simulink library "opm_grc"  (R2024a)
settings: Solver=VariableStepAuto  StartTime=0.0  StopTime=10.0  RelTol=1e-3
undefined symbols (not defined in the file or in its folder): ENUM_IVTROPMODE_ASCLO, ENUM_IVTROPMODE_DTCYCTRL, ENUM_IVTROPMODE_FW, ENUM_IVTROPMODE_IVTROFF, ENUM_MOTMOD_AFTERRUN, ENUM_MOTMOD_DISCHARGE, ENUM_MOTMOD_FAILURE, ENUM_MOTMOD_INIT, ENUM_MOTMOD_READY, ENUM_MOTMOD_SPDCTRL, ENUM_MOTMOD_STANDBY, ENUM_MOTMOD_TQCTROL, GRC_FAKE_SAMPLE_TIME, KOPM_IVTROpMode_enum_ovrdflg, KOPM_IVTROpMode_enum_ovrdval, KOPM_MotMod_enum_ovrdflg, KOPM_MotMod_enum_ovrdval, KOPM_PsvDischrgEna_flg_ovrdflg, KOPM_PsvDischrgEna_flg_ovrdval, OpMod_bDcha2AfterRunMor_C, OpMod_bService_C, OpMod_nRot2AfterRun_C, OpMod_nRotASCDi_C, OpMod_nRotASCEna_C, OpMod_ResolverEnt_C, OpMod_tiDcha2AfterRun_C, OpMod_uDCSide2AfterRun_C
libraries: GRC_Lib x1
settings Model: Creator=FVT22063  LastModifiedBy=FVT22063

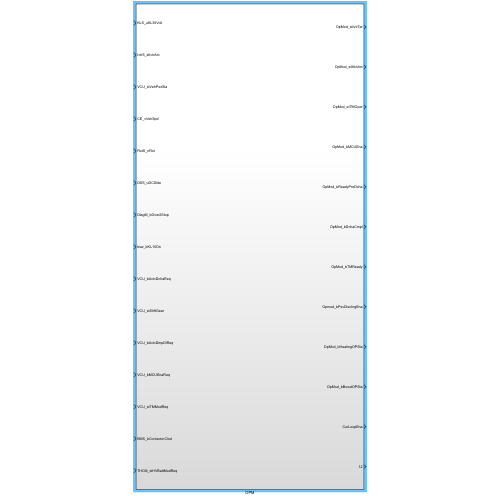
[thumbnail: Simulink's stored preview of the top-level diagram]
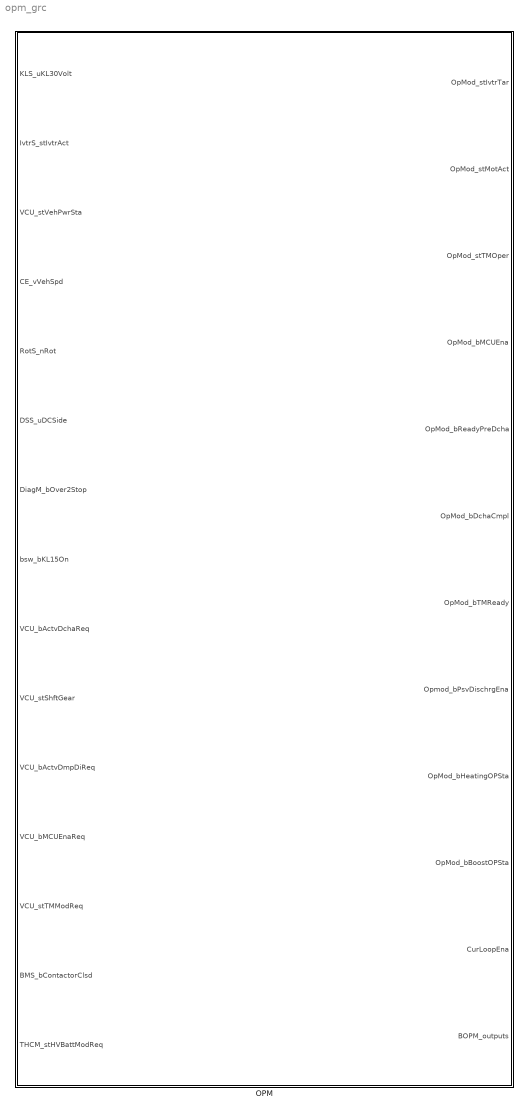
== system opm_grc ==
  OPM : Subsystem

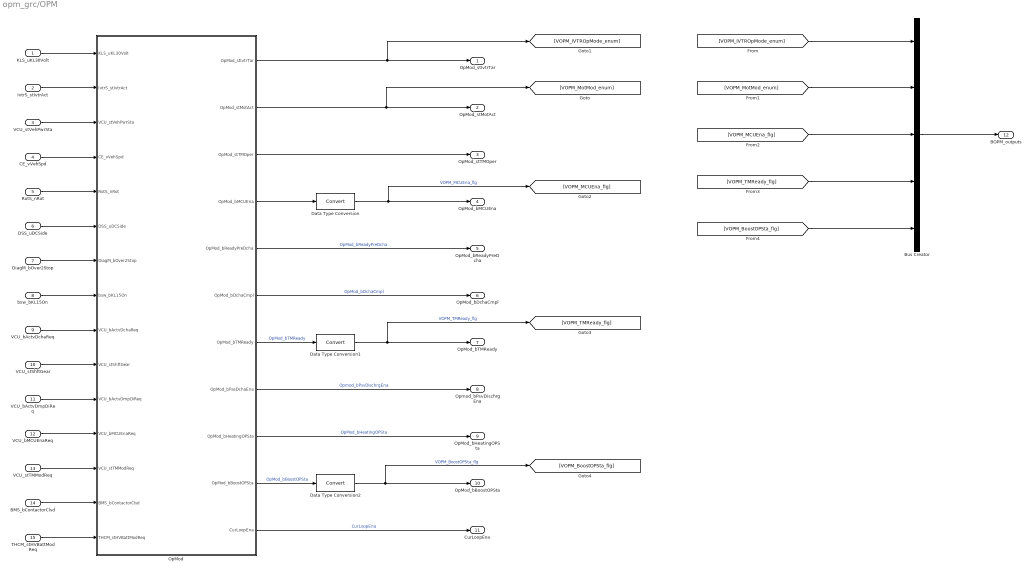
== system opm_grc/OPM ==
  KLS_uKL30Volt : Inport
  IvtrS_stIvtrAct : Inport  Port=2
  VCU_stVehPwrSta : Inport  Port=3
  CE_vVehSpd : Inport  Port=4
  RotS_nRot : Inport  Port=5
  DSS_uDCSide : Inport  Port=6
  DiagM_bOver2Stop : Inport  Port=7
  bsw_bKL15On : Inport  Port=8
  VCU_bActvDchaReq : Inport  Port=9
  VCU_stShftGear : Inport  Port=10
  VCU_bActvDmpDiReq : Inport  Port=11
  VCU_bMCUEnaReq : Inport  Port=12
  VCU_stTMModReq : Inport  Port=13
  BMS_bContactorClsd : Inport  Port=14
  THCM_stHVBattModReq : Inport  Port=15
  Bus Creator : BusCreator  Inputs=5  OutDataTypeStr=Bus: BOPM_outputs  NonVirtualBus=on
  Data Type Conversion : DataTypeConversion  SaturateOnIntegerOverflow=off  RndMeth=Floor
  Data Type Conversion1 : DataTypeConversion  SaturateOnIntegerOverflow=off  RndMeth=Floor
  Data Type Conversion2 : DataTypeConversion  SaturateOnIntegerOverflow=off  RndMeth=Floor
  OpMod : Subsystem  TreatAsAtomicUnit=on
  OpMod_stIvtrTar : Outport
  OpMod_stMotAct : Outport  Port=2
  OpMod_stTMOper : Outport  Port=3
  OpMod_bMCUEna : Outport  Port=4
  OpMod_bReadyPreDcha : Outport  Port=5
  OpMod_bDchaCmpl : Outport  Port=6
  OpMod_bTMReady : Outport  Port=7
  Opmod_bPsvDischrgEna : Outport  Port=8
  OpMod_bHeatingOPSta : Outport  Port=9
  OpMod_bBoostOPSta : Outport  Port=10
  CurLoopEna : Outport  Port=11
  BOPM_outputs : Outport  Port=12  OutDataTypeStr=Bus: BOPM_outputs
  wires:
  RotS_nRot/1 -> OpMod/5(RotS_nRot)
  DSS_uDCSide/1 -> OpMod/6(DSS_uDCSide)
  OpMod/7(OpMod_bTMReady) -> Data Type Conversion1/1  "OpMod_bTMReady"
  VCU_bMCUEnaReq/1 -> OpMod/12(VCU_bMCUEnaReq)
  KLS_uKL30Volt/1 -> OpMod/1(KLS_uKL30Volt)
  THCM_stHVBattModReq/1 -> OpMod/15(THCM_stHVBattModReq)
  CE_vVehSpd/1 -> OpMod/4(CE_vVehSpd)
  OpMod/1(OpMod_stIvtrTar) -> [VOPM_IVTROpMode_enum], OpMod_stIvtrTar/1
  VCU_bActvDchaReq/1 -> OpMod/9(VCU_bActvDchaReq)
  IvtrS_stIvtrAct/1 -> OpMod/2(IvtrS_stIvtrAct)
  DiagM_bOver2Stop/1 -> OpMod/7(DiagM_bOver2Stop)
  VCU_stVehPwrSta/1 -> OpMod/3(VCU_stVehPwrSta)
  bsw_bKL15On/1 -> OpMod/8(bsw_bKL15On)
  OpMod/2(OpMod_stMotAct) -> [VOPM_MotMod_enum], OpMod_stMotAct/1
  VCU_stShftGear/1 -> OpMod/10(VCU_stShftGear)
  OpMod/8(OpMod_bPasDchaEna) -> Opmod_bPsvDischrgEna/1  "Opmod_bPsvDischrgEna"
  VCU_bActvDmpDiReq/1 -> OpMod/11(VCU_bActvDmpDiReq)
  VCU_stTMModReq/1 -> OpMod/13(VCU_stTMModReq)
  BMS_bContactorClsd/1 -> OpMod/14(BMS_bContactorClsd)
  OpMod/3(OpMod_stTMOper) -> OpMod_stTMOper/1
  OpMod/4(OpMod_bMCUEna) -> Data Type Conversion/1
  OpMod/6(OpMod_bDchaCmpl) -> OpMod_bDchaCmpl/1  "OpMod_bDchaCmpl"
  OpMod/5(OpMod_bReadyPreDcha) -> OpMod_bReadyPreDcha/1  "OpMod_bReadyPreDcha"
  OpMod/9(OpMod_bHeatingOPSta) -> OpMod_bHeatingOPSta/1  "OpMod_bHeatingOPSta"
  OpMod/10(OpMod_bBoostOPSta) -> Data Type Conversion2/1  "OpMod_bBoostOPSta"
  OpMod/11(CurLoopEna) -> CurLoopEna/1  "CurLoopEna"
  Data Type Conversion/1 -> [VOPM_MCUEna_flg], OpMod_bMCUEna/1  "VOPM_MCUEna_flg"
  Data Type Conversion1/1 -> [VOPM_TMReady_flg], OpMod_bTMReady/1  "VOPM_TMReady_flg"
  Data Type Conversion2/1 -> [VOPM_BoostOPSta_flg], OpMod_bBoostOPSta/1  "VOPM_BoostOPSta_flg"
  [VOPM_MCUEna_flg] -> Bus Creator/3
  [VOPM_MotMod_enum] -> Bus Creator/2
  [VOPM_IVTROpMode_enum] -> Bus Creator/1
  [VOPM_TMReady_flg] -> Bus Creator/4
  [VOPM_BoostOPSta_flg] -> Bus Creator/5
  Bus Creator/1 -> BOPM_outputs/1

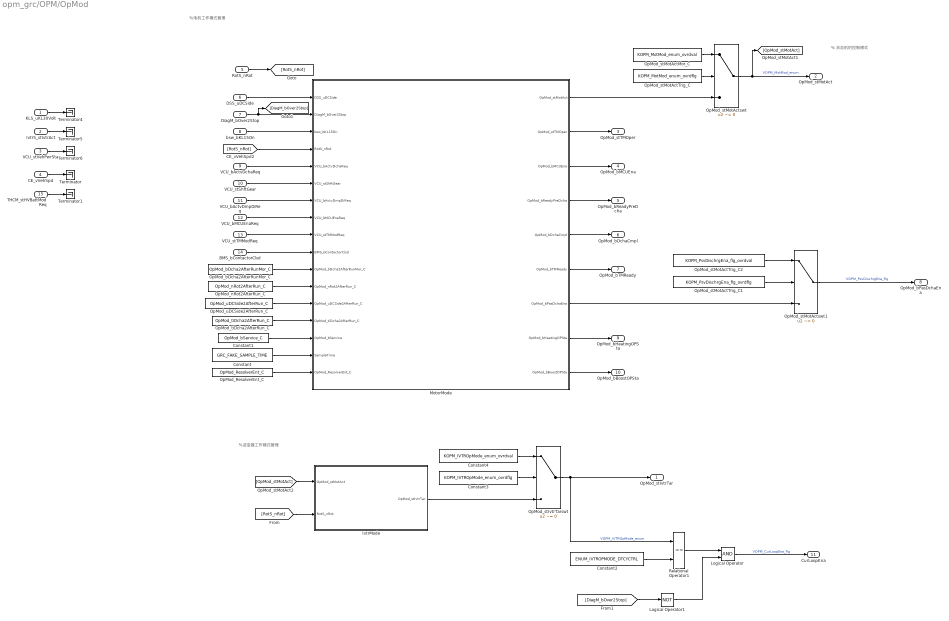
== system opm_grc/OPM/OpMod ==
  note: % 状态机的控制模式
  note: %电机工作模式管理
  note: %逆变器工作模式管理
  KLS_uKL30Volt : Inport
  IvtrS_stIvtrAct : Inport  Port=2
  VCU_stVehPwrSta : Inport  Port=3
  CE_vVehSpd : Inport  Port=4
  RotS_nRot : Inport  Port=5  OutDataTypeStr=single
  DSS_uDCSide : Inport  Port=6
  DiagM_bOver2Stop : Inport  Port=7
  bsw_bKL15On : Inport  Port=8
  VCU_bActvDchaReq : Inport  Port=9
  VCU_stShftGear : Inport  Port=10
  VCU_bActvDmpDiReq : Inport  Port=11
  VCU_bMCUEnaReq : Inport  Port=12
  VCU_stTMModReq : Inport  Port=13
  BMS_bContactorClsd : Inport  Port=14
  THCM_stHVBattModReq : Inport  Port=15
  Constant : Constant  Value=GRC_FAKE_SAMPLE_TIME
  Constant1 : Constant  Value=OpMod_bService_C
  Constant2 : Constant  Value=ENUM_IVTROPMODE_DTCYCTRL
  Constant3 : Constant  Value=KOPM_IVTROpMode_enum_ovrdflg
  Constant4 : Constant  Value=KOPM_IVTROpMode_enum_ovrdval
  IvtrMode : Subsystem
  Logical Operator : Logic  AllPortsSameDT=off  OutDataTypeStr=boolean
  Logical Operator1 : Logic  Operator=NOT  AllPortsSameDT=off  OutDataTypeStr=boolean
  MotorMode : Stateflow chart  TreatAsAtomicUnit=on
  OpMod_ResolverEnt_C : Constant  Value=OpMod_ResolverEnt_C
  OpMod_bDcha2AfterRunMor_C : Constant  Value=OpMod_bDcha2AfterRunMor_C  OutMin=0  OutMax=1
  OpMod_nRot2AfterRun_C : Constant  Value=OpMod_nRot2AfterRun_C
  OpMod_stIvtrTarswt : Switch  Criteria=u2 ~= 0  SaturateOnIntegerOverflow=off  InputSameDT=off
  OpMod_stMotActMor_C : Constant  Value=KOPM_MotMod_enum_ovrdval
  OpMod_stMotActTrig_C : Constant  Value=KOPM_MotMod_enum_ovrdflg
  OpMod_stMotActTrig_C1 : Constant  Value=KOPM_PsvDischrgEna_flg_ovrdflg
  OpMod_stMotActTrig_C2 : Constant  Value=KOPM_PsvDischrgEna_flg_ovrdval
  OpMod_stMotActswt : Switch  Criteria=u2 ~= 0  SaturateOnIntegerOverflow=off  InputSameDT=off
  OpMod_stMotActswt1 : Switch  Criteria=u2 ~= 0  SaturateOnIntegerOverflow=off  InputSameDT=off
  OpMod_tiDcha2AfterRun_C : Constant  Value=OpMod_tiDcha2AfterRun_C
  OpMod_uDCSide2AfterRun_C : Constant  Value=OpMod_uDCSide2AfterRun_C
  Relational Operator1 : RelationalOperator  Operator===  OutDataTypeStr=boolean  RndMeth=Simplest  InputSameDT=off
  Terminator{,1,4..6} (5 alike) : Terminator
  OpMod_stIvtrTar : Outport  VectorParamsAs1DForOutWhenUnconnected=off
  OpMod_stMotAct : Outport  Port=2  VectorParamsAs1DForOutWhenUnconnected=off
  OpMod_stTMOper : Outport  Port=3  VectorParamsAs1DForOutWhenUnconnected=off
  OpMod_bMCUEna : Outport  Port=4  VectorParamsAs1DForOutWhenUnconnected=off
  OpMod_bReadyPreDcha : Outport  Port=5  VectorParamsAs1DForOutWhenUnconnected=off
  OpMod_bDchaCmpl : Outport  Port=6  VectorParamsAs1DForOutWhenUnconnected=off
  OpMod_bTMReady : Outport  Port=7  VectorParamsAs1DForOutWhenUnconnected=off
  OpMod_bPasDchaEna : Outport  Port=8  VectorParamsAs1DForOutWhenUnconnected=off
  OpMod_bHeatingOPSta : Outport  Port=9  VectorParamsAs1DForOutWhenUnconnected=off
  OpMod_bBoostOPSta : Outport  Port=10  VectorParamsAs1DForOutWhenUnconnected=off
  CurLoopEna : Outport  Port=11
  wires:
  Constant4/1 -> OpMod_stIvtrTarswt/1
  Constant3/1 -> OpMod_stIvtrTarswt/2
  KLS_uKL30Volt/1 -> Terminator4/1
  CE_vVehSpd/1 -> Terminator/1
  VCU_stVehPwrSta/1 -> Terminator6/1
  IvtrS_stIvtrAct/1 -> Terminator5/1
  [OpMod_stMotAct] -> IvtrMode/1(OpMod_stMotAct)
  [RotS_nRot] -> IvtrMode/2(RotS_nRot)
  IvtrMode/1(OpMod_stIvtrTar) -> OpMod_stIvtrTarswt/3
  DiagM_bOver2Stop/1 -> [DiagM_bOver2Stop], MotorMode/2(DiagM_bOver2Stop)
  OpMod_stMotActswt/1 -> [OpMod_stMotAct], OpMod_stMotAct/1  "VOPM_MotMod_enum"
  OpMod_stMotActMor_C/1 -> OpMod_stMotActswt/1
  OpMod_stMotActTrig_C/1 -> OpMod_stMotActswt/2
  VCU_bMCUEnaReq/1 -> MotorMode/8(VCU_bMCUEnaReq)
  Constant/1 -> MotorMode/16(SampleTime)
  OpMod_tiDcha2AfterRun_C/1 -> MotorMode/14(OpMod_tiDcha2AfterRun_C)
  MotorMode/2(OpMod_stTMOper) -> OpMod_stTMOper/1
  OpMod_uDCSide2AfterRun_C/1 -> MotorMode/13(OpMod_uDCSide2AfterRun_C)
  OpMod_nRot2AfterRun_C/1 -> MotorMode/12(OpMod_nRot2AfterRun_C)
  MotorMode/6(OpMod_bTMReady) -> OpMod_bTMReady/1
  MotorMode/5(OpMod_bDchaCmpl) -> OpMod_bDchaCmpl/1
  Constant1/1 -> MotorMode/15(OpMod_bService)
  MotorMode/4(OpMod_bReadyPreDcha) -> OpMod_bReadyPreDcha/1
  OpMod_bDcha2AfterRunMor_C/1 -> MotorMode/11(OpMod_bDcha2AfterRunMor_C)
  MotorMode/8(OpMod_bHeatingOPSta) -> OpMod_bHeatingOPSta/1
  MotorMode/3(OpMod_bMCUEna) -> OpMod_bMCUEna/1
  RotS_nRot/1 -> [RotS_nRot]
  VCU_bActvDchaReq/1 -> MotorMode/5(VCU_bActvDchaReq)
  VCU_stShftGear/1 -> MotorMode/6(VCU_stShftGear)
  MotorMode/9(OpMod_bBoostOPSta) -> OpMod_bBoostOPSta/1
  VCU_stTMModReq/1 -> MotorMode/9(VCU_stTMModReq)
  [RotS_nRot] -> MotorMode/4(RotS_nRot)
  MotorMode/7(OpMod_bPasDchaEna) -> OpMod_stMotActswt1/3
  bsw_bKL15On/1 -> MotorMode/3(bsw_bKL15On)
  BMS_bContactorClsd/1 -> MotorMode/10(BMS_bContactorClsd)
  MotorMode/1(OpMod_stMotAct) -> OpMod_stMotActswt/3
  VCU_bActvDmpDiReq/1 -> MotorMode/7(VCU_bActvDmpDiReq)
  DSS_uDCSide/1 -> MotorMode/1(DSS_uDCSide)
  OpMod_ResolverEnt_C/1 -> MotorMode/17(OpMod_ResolverEnt_C)
  OpMod_stMotActswt1/1 -> OpMod_bPasDchaEna/1  "VOPM_PsvDischrgEna_flg"
  OpMod_stMotActTrig_C1/1 -> OpMod_stMotActswt1/2
  OpMod_stMotActTrig_C2/1 -> OpMod_stMotActswt1/1
  THCM_stHVBattModReq/1 -> Terminator1/1
  OpMod_stIvtrTarswt/1 -> Relational Operator1/1, OpMod_stIvtrTar/1  "VOPM_IVTROpMode_enum"
  Constant2/1 -> Relational Operator1/2
  Logical Operator/1 -> CurLoopEna/1  "VOPM_CurLoopEna_flg"
  [DiagM_bOver2Stop] -> Logical Operator1/1
  Logical Operator1/1 -> Logical Operator/2
  Relational Operator1/1 -> Logical Operator/1

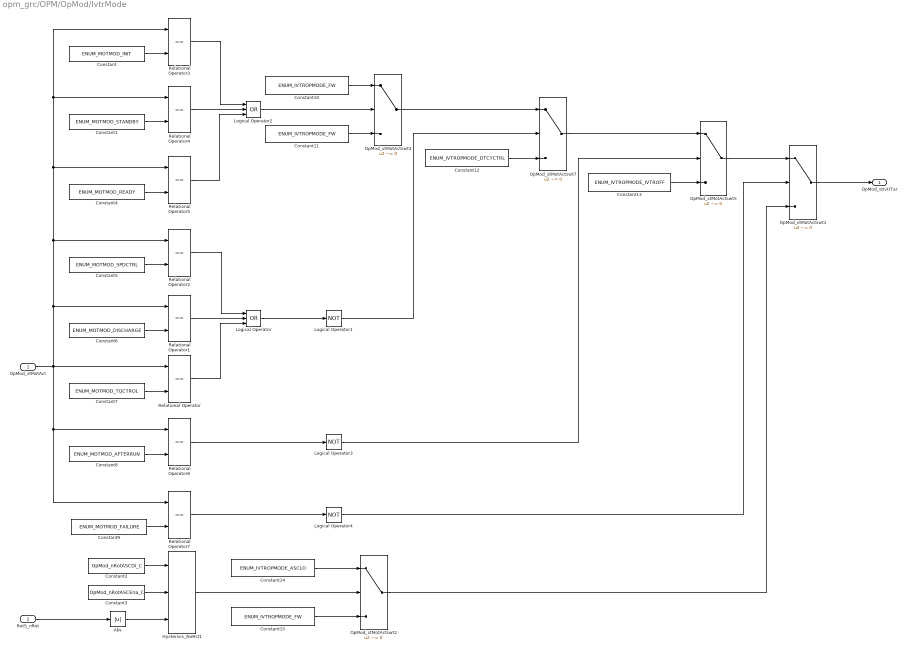
== system opm_grc/OPM/OpMod/IvtrMode ==
  OpMod_stMotAct : Inport
  RotS_nRot : Inport  Port=2  OutDataTypeStr=single
  Abs : Abs  SaturateOnIntegerOverflow=off
  Constant : Constant  Value=ENUM_MOTMOD_INIT
  Constant1 : Constant  Value=ENUM_MOTMOD_STANDBY
  Constant10 : Constant  Value=ENUM_IVTROPMODE_FW
  Constant11 : Constant  Value=ENUM_IVTROPMODE_FW
  Constant12 : Constant  Value=ENUM_IVTROPMODE_DTCYCTRL
  Constant13 : Constant  Value=ENUM_IVTROPMODE_IVTROFF
  Constant14 : Constant  Value=ENUM_IVTROPMODE_ASCLO
  Constant15 : Constant  Value=ENUM_IVTROPMODE_FW
  Constant2 : Constant  Value=OpMod_nRotASCDi_C
  Constant3 : Constant  Value=OpMod_nRotASCEna_C
  Constant4 : Constant  Value=ENUM_MOTMOD_READY
  Constant5 : Constant  Value=ENUM_MOTMOD_SPDCTRL
  Constant6 : Constant  Value=ENUM_MOTMOD_DISCHARGE
  Constant7 : Constant  Value=ENUM_MOTMOD_TQCTROL
  Constant8 : Constant  Value=ENUM_MOTMOD_AFTERRUN
  Constant9 : Constant  Value=ENUM_MOTMOD_FAILURE
  Hysterisis_NoRst1 : GRC_Lib/Nonlinear/Hysterisis_NoRst  SystemSampleTime=-1  VariantActivationTime=update diagram  AllowFlexibleInterface=on  Latency=0  AutoFrameSizeCalculation=off
  Logical Operator : Logic  Operator=OR  Inputs=3  AllPortsSameDT=off  OutDataTypeStr=boolean
  Logical Operator1 : Logic  Operator=NOT  AllPortsSameDT=off  OutDataTypeStr=boolean
  Logical Operator2 : Logic  Operator=OR  Inputs=3  AllPortsSameDT=off  OutDataTypeStr=boolean
  Logical Operator3 : Logic  Operator=NOT  AllPortsSameDT=off  OutDataTypeStr=boolean
  Logical Operator4 : Logic  Operator=NOT  AllPortsSameDT=off  OutDataTypeStr=boolean
  OpMod_stMotActswt{1..2,4..5,7} (5 alike) : Switch  Criteria=u2 ~= 0  SaturateOnIntegerOverflow=off  InputSameDT=off
  Relational Operator{,1..7} (8 alike) : RelationalOperator  Operator===  OutDataTypeStr=boolean  RndMeth=Simplest  InputSameDT=off
  OpMod_stIvtrTar : Outport  VectorParamsAs1DForOutWhenUnconnected=off
  wires:
  Relational Operator/1 -> Logical Operator/3
  Constant7/1 -> Relational Operator/2
  RotS_nRot/1 -> Abs/1
  Constant3/1 -> Hysterisis_NoRst1/2
  Constant2/1 -> Hysterisis_NoRst1/1
  Abs/1 -> Hysterisis_NoRst1/3
  Constant6/1 -> Relational Operator1/2
  Relational Operator1/1 -> Logical Operator/2
  Constant5/1 -> Relational Operator2/2
  Relational Operator2/1 -> Logical Operator/1
  Constant/1 -> Relational Operator3/2
  Constant1/1 -> Relational Operator4/2
  Constant4/1 -> Relational Operator5/2
  Relational Operator5/1 -> Logical Operator2/3
  Relational Operator4/1 -> Logical Operator2/2
  Relational Operator3/1 -> Logical Operator2/1
  Logical Operator2/1 -> OpMod_stMotActswt4/2
  Constant11/1 -> OpMod_stMotActswt4/3
  Constant8/1 -> Relational Operator6/2
  OpMod_stMotAct/1 -> Relational Operator7/1, Relational Operator6/1, Relational Operator/1, Relational Operator3/1, Relational Operator4/1, Relational Operator5/1, Relational Operator2/1, Relational Operator1/1
  Constant12/1 -> OpMod_stMotActswt7/3
  Logical Operator/1 -> Logical Operator1/1
  OpMod_stMotActswt4/1 -> OpMod_stMotActswt7/1
  Relational Operator6/1 -> Logical Operator3/1
  OpMod_stMotActswt7/1 -> OpMod_stMotActswt5/1
  Constant13/1 -> OpMod_stMotActswt5/3
  OpMod_stMotActswt5/1 -> OpMod_stMotActswt1/1
  OpMod_stMotActswt1/1 -> OpMod_stIvtrTar/1
  Constant10/1 -> OpMod_stMotActswt4/1
  Constant9/1 -> Relational Operator7/2
  Hysterisis_NoRst1/1 -> OpMod_stMotActswt2/2
  Relational Operator7/1 -> Logical Operator4/1
  Constant14/1 -> OpMod_stMotActswt2/1
  Constant15/1 -> OpMod_stMotActswt2/3
  OpMod_stMotActswt2/1 -> OpMod_stMotActswt1/3
  Logical Operator1/1 -> OpMod_stMotActswt7/2
  Logical Operator3/1 -> OpMod_stMotActswt5/2
  Logical Operator4/1 -> OpMod_stMotActswt1/2

== stateflow chart opm_grc/OPM/OpMod/MotorMode ==
  state MotStM
    state PowerDownProcedure
      state PowerUpProcedure
        state Initial
          en:
          OpMod_stMotAct = ENUM_MOTMOD_INIT;
        state StandBy
          en:
          OpMod_stMotAct = ENUM_MOTMOD_STANDBY;
          OpMod_bReadyPreDcha = 1;
        state Ready
          en:
          OpMod_stMotAct = ENUM_MOTMOD_READY;
          OpMod_bTMReady = 1;
        state Torque
          en:
          OpMod_stMotAct = ENUM_MOTMOD_TQCTROL;
          OpMod_bMCUEna = 1;
          OpMod_stTMOper = 0;
        state Speed
          en:
          OpMod_stMotAct = ENUM_MOTMOD_SPDCTRL;
          OpMod_bMCUEna = 1;
          OpMod_stTMOper = 1;
        state Heating
          en:
          OpMod_stMotAct = ENUM_MOTMOD_HEATING;
          OpMod_bHeatingOPSta = 1;
        state Boosting
          en:
          OpMod_stMotAct = ENUM_MOTMOD_BOOSTCHRG;
          OpMod_bBoostOPSta = 1;
        state ResolverAdjust
          en:
          OpMod_stMotAct = ENUM_MOTMOD_RESOLVERADJUST;
        state DiagService
          en:
          OpMod_stMotAct = ENUM_MOTMOD_DIAGSERV;
        (default) -> Initial
        Initial -> StandBy : [bsw_bKL15On == 1]
        StandBy -> Ready : [BMS_bContactorClsd == 1 && DSS_uDCSide > OpMod_uDCSide2AfterRun_C]
        (junction 267) -> Ready
        (junction 268) -> (junction 267)
        Ready -> (junction 269)
        (junction 269) -> Torque [order 1] : [VCU_bMCUEnaReq == 1 &&...
            | VCU_stTMModReq == ENUM_CTRLMODE_TQMODE &&...
            | VCU_stShftGear ~= ENUM_GEARPOSN_PARK &&...
            | VCU_bActvDmpDiReq == 1]
        (junction 269) -> (junction 270) [order 2]
        Torque -> (junction 268) [order 2] : [VCU_bMCUEnaReq ~= 1 ||...
            | VCU_stShftGear == ENUM_GEARPOSN_PARK  ||...
            | VCU_bActvDmpDiReq ~= 1]
        (junction 256) -> (junction 268)
        Torque -> Speed [order 1] : [VCU_stTMModReq == ENUM_CTRLMODE_SPDMODE]
        Speed -> Torque [order 1] : [VCU_stTMModReq == ENUM_CTRLMODE_TQMODE]
        (junction 270) -> Speed [order 1] : [VCU_bMCUEnaReq == 1 &&...
            | VCU_stTMModReq == ENUM_CTRLMODE_SPDMODE &&...
            | VCU_stShftGear ~= ENUM_GEARPOSN_PARK &&...
            | VCU_bActvDmpDiReq == 1]
        (junction 270) -> (junction 272) [order 2]
        Speed -> (junction 256) [order 2] : [VCU_bMCUEnaReq ~= 1 ||...
            | VCU_stShftGear == ENUM_GEARPOSN_PARK  ||...
            | VCU_bActvDmpDiReq ~= 1]
        (junction 271) -> (junction 256)
        (junction 272) -> Heating [order 1] : [VCU_bMCUEnaReq == 0 &&...
            | VCU_stTMModReq == ENUM_CTRLMODE_HEATGMOD &&...
            | VCU_stShftGear == ENUM_GEARPOSN_PARK]
        Heating -> (junction 271) : [VCU_bMCUEnaReq ~= 0 ||...
            | VCU_stTMModReq ~= ENUM_CTRLMODE_HEATGMOD ||...
            | VCU_stShftGear ~= ENUM_GEARPOSN_PARK ]
        (junction 272) -> (junction 257) [order 2]
        (junction 273) -> (junction 271)
        (junction 257) -> Boosting [order 1] : [VCU_bMCUEnaReq == 0 &&...
            | VCU_stTMModReq == ENUM_CTRLMODE_BOOSTMOD &&...
            | VCU_stShftGear == ENUM_GEARPOSN_PARK]
        Boosting -> (junction 273) : [VCU_bMCUEnaReq ~= 0 ||...
            | VCU_stTMModReq ~= ENUM_CTRLMODE_BOOSTMOD ||...
            | VCU_stShftGear ~= ENUM_GEARPOSN_PARK ]
        (junction 257) -> (junction 552) [order 2]
        (junction 557) -> (junction 273)
        ResolverAdjust -> (junction 557) : [OpMod_ResolverEnt_C == 0]
        (junction 552) -> ResolverAdjust [order 1] : [OpMod_ResolverEnt_C == 1]
        (junction 566) -> (junction 557)
        (junction 552) -> (junction 561) [order 2]
        (junction 561) -> DiagService : [OpMod_bService == 1]
        DiagService -> (junction 566) : [OpMod_bService == 0]
      state FailureMode
        en:
        OpMod_stMotAct = ENUM_MOTMOD_FAILURE;
      (default) -> PowerUpProcedure
      PowerUpProcedure -> FailureMode : [DiagM_bOver2Stop == 1]
    state DischargeMode
      en:
      OpMod_stMotAct = ENUM_MOTMOD_DISCHARGE;
      OpMod_DchaTmr = 0;
      du:
      OpMod_DchaTmr = OpMod_DchaTmr + SampleTime;
    (default) -> PowerDownProcedure
    PowerDownProcedure -> DischargeMode : [VCU_bActvDchaReq == 1 &&...
        | BMS_bContactorClsd == 0 &&...
        | DiagM_bOver2Stop == 0]
    DischargeMode -> FailureMode : [DiagM_bOver2Stop == 1]{OpMod_bPasDchaEna = 1}
  note: % 需要底层发送一个网络休眠标志位
  state AfterRunMode
    en:
    OpMod_bPasDchaEna = 0;
    OpMod_stMotAct = ENUM_MOTMOD_AFTERRUN;
    du:
    AfterRunChoice((DSS_uDCSide < OpMod_uDCSide2AfterRun_C) || (OpMod_bDcha == OpMod_bDcha2AfterRunMor_C));
  state AfterRunChoice (choice) [function]
    (default) -> (junction 507)
    (junction 507) -> (junction 511) [order 1] : [choice]
    (junction 507) -> (junction 505) [order 2] : {OpMod_bDchaCmpl = 0;}
    (junction 511) -> (junction 508) : {OpMod_bDchaCmpl = 1;}
    (junction 508) -> (junction 505)
    (junction 505) -> (junction 503)
  (default) -> MotStM
  AfterRunMode -> StandBy : [bsw_bKL15On == 1 &&...
      | DiagM_bOver2Stop == 0]
  MotStM -> AfterRunMode [order 1] : [bsw_bKL15On == 0 &&...
      | OpMod_DchaTmr > OpMod_tiDcha2AfterRun_C &&...
      | RotS_nRot < OpMod_nRot2AfterRun_C]
  MotStM -> AfterRunMode [order 2] : [bsw_bKL15On == 0 &&...
      | DSS_uDCSide < OpMod_uDCSide2AfterRun_C &&...
      | RotS_nRot < OpMod_nRot2AfterRun_C]
  data: choice function_input double; DSS_uDCSide input single size=1; OpMod_stMotAct output uint8 size=1; DiagM_bOver2Stop input boolean size=1; bsw_bKL15On input boolean size=1; RotS_nRot input single size=1; VCU_bActvDchaReq input boolean size=1; VCU_stShftGear input uint8 size=1; VCU_bActvDmpDiReq input boolean size=1; VCU_bMCUEnaReq input boolean size=1; VCU_stTMModReq input uint8 size=1; BMS_bContactorClsd input boolean size=1; OpMod_stTMOper output uint8 size=1; OpMod_bDcha2AfterRunMor_C input; OpMod_bMCUEna output boolean size=1; OpMod_bReadyPreDcha output boolean size=1; OpMod_bDchaCmpl output boolean size=1; OpMod_bTMReady output boolean size=1; OpMod_bPasDchaEna output boolean size=1; OpMod_bHeatingOPSta output boolean size=1; OpMod_bBoostOPSta output boolean size=1; OpMod_nRot2AfterRun_C input; OpMod_uDCSide2AfterRun_C input; OpMod_tiDcha2AfterRun_C input; OpMod_bService input; SampleTime input; OpMod_DchaTmr local single; OpMod_bDcha local boolean; OpMod_ResolverEnt_C input; ENUM_MOTMOD_INIT parameter; ENUM_MOTMOD_READY parameter; ENUM_MOTMOD_RESOLVERADJUST parameter; ENUM_MOTMOD_SPDCTRL parameter; ENUM_MOTMOD_STANDBY parameter; ENUM_MOTMOD_TQCTROL parameter; ENUM_GEARPOSN_PARK parameter; ENUM_MOTMOD_AFTERRUN parameter; ENUM_MOTMOD_BOOSTCHRG parameter; ENUM_MOTMOD_DIAGSERV parameter; ENUM_MOTMOD_DISCHARGE parameter; ENUM_MOTMOD_FAILURE parameter; ENUM_MOTMOD_HEATING parameter; ENUM_CTRLMODE_BOOSTMOD parameter; ENUM_CTRLMODE_HEATGMOD parameter; ENUM_CTRLMODE_SPDMODE parameter; ENUM_CTRLMODE_TQMODE parameter
